simulink model "Vdq_response"  (Simulink 8.1)
settings: Solver=ode23t  StartTime=0.0  StopTime=0.5  MaxStep=25e-6  RelTol=1e-3  AbsTol=1e-4
undefined symbols (not defined in the file or in its folder): tf_cl
libraries: cstblocks x4, simulink x1, powerlib x1
settings Model: Creator=marko  LastModifiedBy=wenbo  BufferReuse=off
settings OptimizationCC: BlockReduction=off  InlineParams=on  BufferReuse=off
settings DebuggingCC: AlgebraicLoopMsg=none  SolverPrmCheckMsg=none  FcnCallInpInsideContextMsg=EnableAllAsWarning  UnconnectedInputMsg=none  UnconnectedOutputMsg=none  UnconnectedLineMsg=none  StrictBusMsg=Warning
settings ConfigurationSet: Description=SimMechanics 2G

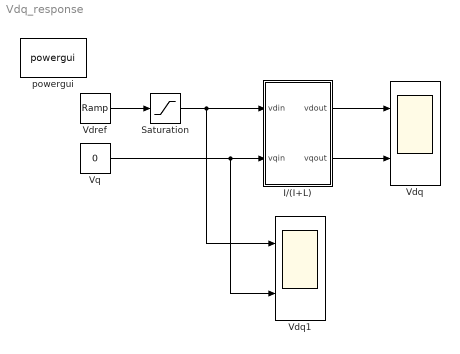
== system Vdq_response ==
  I/(I+L) : Subsystem
  Saturation : Saturate  UpperLimit=99.6  LowerLimit=0
  Vdq : Scope  NumInputPorts=2
      settings: YMin=0~-7.5  YMax=120~20  SaveName=Vdq_sim
  Vdq1 : Scope  NumInputPorts=2
      settings: TimeRange=0.05  YMin=50~-1  YMax=100~1
  Vdref : simulink/Sources/Ramp  slope=5000  start=0  X0=0
  Vq : Constant  Value=0
  powergui : powerlib/powergui  Priority=1  SimulationMode=Continuous  SolverType=Tustin  SampleTime=50e-6  frequency=60  SPID=off  DisableSnubberDevices=off  DisableRonSwitches=off  DisableVfSwitches=off  SwTol=0  Interpol=off  DisplayEquations=off  frequencyindice=0  Pbase=100e6  ErrMax=1e-4  Iterations=50  UnitsV=kV  UnitsW=MW  FunctionMessages=off  echomessages=off  HookPort=off  EnableUseOfTLC=off  x0status=blocks  RestoreLinks=warning  ResistiveCurrentMeasurement=off  Frange=[0:2:500]  Ylog=off  Xlog=on  ShowGrid=off  save=off  variable=ZData  ZoomFFT=on  StartTime=0.0  cycles=1  DisplayStyle=1  fundamental=60  FreqAxis=off  MaxFrequency=1000  frequencyindicesteady=1  RmsSteady=1  display=off  Ts=0  methode=off
  wires:
  Vdref/1 -> Saturation/1
  Saturation/1 -> Vdq1/1, I/(I+L)/1(vdin)
  Vq/1 -> Vdq1/2, I/(I+L)/2(vqin)
  I/(I+L)/2(vqout) -> Vdq/2
  I/(I+L)/1(vdout) -> Vdq/1

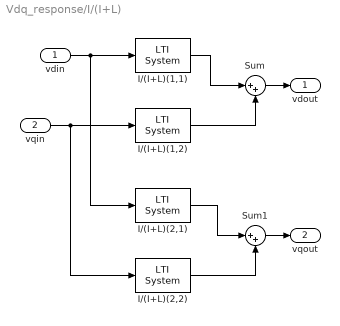
== system Vdq_response/I/(I+L) ==
  vdin : Inport
  vqin : Inport  Port=2
  I/(I+L)(1,1) : cstblocks/LTI System  sys=tf_cl(1,1)  IC=[]
  I/(I+L)(1,2) : cstblocks/LTI System  sys=tf_cl(1,2)  IC=[]
  I/(I+L)(2,1) : cstblocks/LTI System  sys=tf_cl(2,1)  IC=[]
  I/(I+L)(2,2) : cstblocks/LTI System  sys=tf_cl(2,2)  IC=[]
  Sum : Sum  Inputs=|++
  Sum1 : Sum  Inputs=|++
  vdout : Outport
  vqout : Outport  Port=2
  wires:
  I/(I+L)(1,1)/1 -> Sum/1
  I/(I+L)(2,2)/1 -> Sum1/2
  vdin/1 -> I/(I+L)(1,1)/1, I/(I+L)(2,1)/1
  vqin/1 -> I/(I+L)(1,2)/1, I/(I+L)(2,2)/1
  Sum/1 -> vdout/1
  Sum1/1 -> vqout/1
  I/(I+L)(1,2)/1 -> Sum/2
  I/(I+L)(2,1)/1 -> Sum1/1
